simulink model "sim01"  (R2020a)
settings: Solver=VariableStepAuto  StartTime=0.0  StopTime=10.0  RelTol=1e-3
values from neighbouring files (symbols this model uses):
  Cp = 1000    [lab01.m]    (also in skrypt.m; sprawozdanie.m)
  Cv1 = Cp*Pp*V1    (= 108000)    [lab01.m]    (also in skrypt.m; sprawozdanie.m)
  Cv2 = Cp*Pp*V2    (= 144000)    [lab01.m]    (also in skrypt.m; sprawozdanie.m)
  czas_skoku = 40    [lab01.m]    (also in sprawozdanie.m = 60)
  dufp = 0    [lab01.m]    (also in sprawozdanie.m)
  duTkz = 0    [lab01.m]    (also in sprawozdanie.m)
  duTzew = 0    [lab01.m]    (also in sprawozdanie.m)
  fp = Tab_fp(i)    [lab01.m]    (also in skrypt.m = Tab_fp(j); sprawozdanie.m = 0.25)
  Ko = (qkN-Ks*(Tw1N-TzewN))/(Tw1N-Tw2N)    (= 240)    [lab01.m]    (also in skrypt.m; sprawozdanie.m)
  Ks = (Cp*Pp*fpN*(TkzN-Tw2N))/(Tw1N+Tw2N-2*TzewN)    (= 120)    [lab01.m]    (also in skrypt.m; sprawozdanie.m)
  Pp = 1.2    [lab01.m]    (also in skrypt.m; sprawozdanie.m)
  Tkz = Tab_Tkz(i)    [lab01.m]    (also in skrypt.m; sprawozdanie.m)
  Tw10 = ((Ko+Ks+Cp*Pp*fp)*(Cp*Pp*Tkz*fp+Ks*Tzew)+Ko*Ks*Tzew)/((Cp*Pp*fp+Ks+Ko)^2-Ko*(Ko+Cp*Pp*fp))    [lab01.m]    (also in sprawozdanie.m)
  Tw20 = (Tw10*(Ko+Cp*Pp*fp)+Ks*Tzew)/(Ko+Ks+Cp*Pp*fp)    [lab01.m]    (also in sprawozdanie.m)
  Tzew = Tab_Tzew(i)    [lab01.m]    (also in skrypt.m; sprawozdanie.m)
settings Model: Creator=jakub  LastModifiedBy=jakub

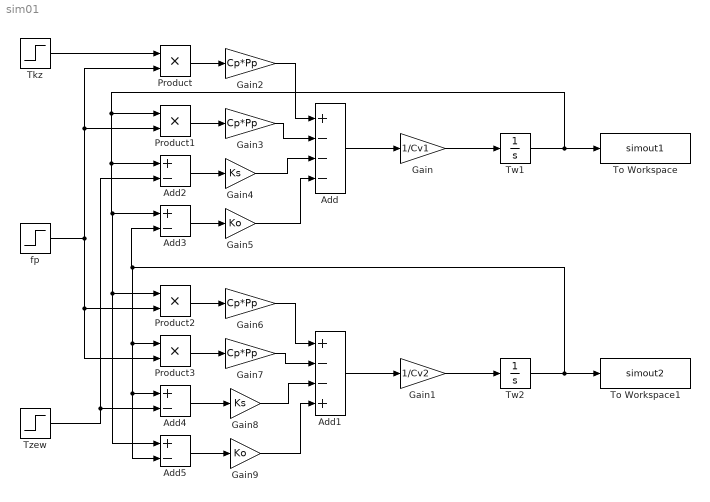
== system sim01 ==
  Add : Sum  Inputs=+---
  Add1 : Sum  Inputs=+--+
  Add{2..5} (4 alike) : Sum  Inputs=+-
  Gain : Gain  Gain=1/Cv1
  Gain1 : Gain  Gain=1/Cv2
  Gain{2..3,6..7} (4 alike) : Gain  Gain=Cp*Pp
  Gain4 : Gain  Gain=Ks
  Gain5 : Gain  Gain=Ko
  Gain8 : Gain  Gain=Ks
  Gain9 : Gain  Gain=Ko
  Product{,1..3} (4 alike) : Product
  Tkz : Step  Time=czas_skoku  Before=Tkz  After=Tkz+duTkz  SampleTime=0
  To Workspace : ToWorkspace  VariableName=simout1  SampleTime=-1
  To Workspace1 : ToWorkspace  VariableName=simout2  SampleTime=-1
  Tw1 : Integrator  InitialCondition=Tw10
  Tw2 : Integrator  InitialCondition=Tw20
  Tzew : Step  Time=czas_skoku  Before=Tzew  After=Tzew+duTzew  SampleTime=0
  fp : Step  Time=czas_skoku  Before=fp  After=fp+dufp  SampleTime=0
  wires:
  Tw1/1 -> Add5/1, Product2/1, Add3/1, Add2/1, Product1/1, To Workspace/1
  Gain1/1 -> Tw2/1
  Gain/1 -> Tw1/1
  Add1/1 -> Gain1/1
  Add/1 -> Gain/1
  Tkz/1 -> Product/1
  fp/1 -> Product1/2, Product/2, Product3/2, Product2/2
  Product/1 -> Gain2/1
  Product1/1 -> Gain3/1
  Gain2/1 -> Add/1
  Gain3/1 -> Add/2
  Add2/1 -> Gain4/1
  Gain4/1 -> Add/3
  Tzew/1 -> Add4/2, Add2/2
  Add3/1 -> Gain5/1
  Gain5/1 -> Add/4
  Gain6/1 -> Add1/1
  Product2/1 -> Gain6/1
  Tw2/1 -> Add5/2, Add4/1, Product3/1, Add3/2, To Workspace1/1
  Gain7/1 -> Add1/2
  Product3/1 -> Gain7/1
  Gain8/1 -> Add1/3
  Add4/1 -> Gain8/1
  Add5/1 -> Gain9/1
  Gain9/1 -> Add1/4
